simulink subsystem "sm_rc_initializer"  (R2023a)
settings: Solver=VariableStepAuto  StartTime=0.0  StopTime=10.0  RelTol=1e-3
settings Model: Creator=thesa  LastModifiedBy=thesa

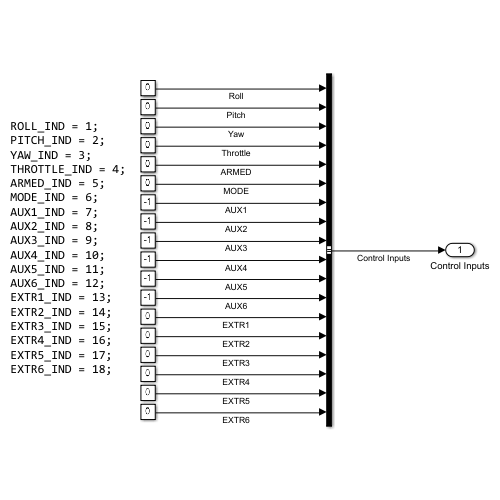
[thumbnail: Simulink's stored preview of the top-level diagram]
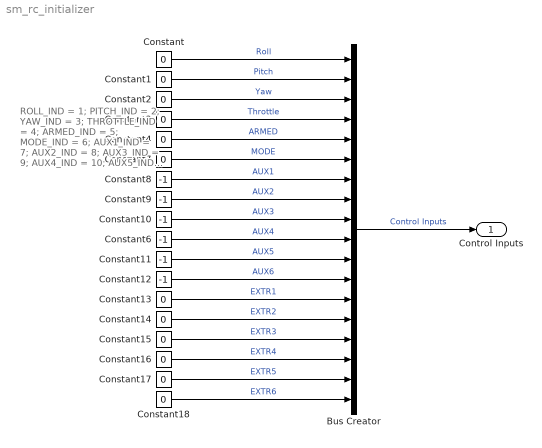
== system sm_rc_initializer ==
  note: ROLL_IND = 1;
      | PITCH_IND = 2;
      | YAW_IND = 3;
      | THROTTLE_IND = 4;
      | ARMED_IND = 5;
      | MODE_IND = 6;
      | AUX1_IND = 7;
      | AUX2_IND = 8;
      | AUX3_IND = 9;
      | AUX4_IND = 10;
      | AUX5_IND = 11;
      | AUX6_IND = 12;
      | EXTR1_IND = 13;
      | EXTR2_IND = 14;
      | EXTR3_IND = 15;
      | EXTR4_IND = 16;
      | EXTR5_IND = 17;
      | EXTR6_IND = 18;
  Bus Creator : BusCreator  Inputs=18
  Constant{,1..4,7,13..18} (12 alike) : Constant  Value=0
  Constant{6,8..12} (6 alike) : Constant  Value=-1
  Control Inputs : Outport
  wires:
  Constant12/1 -> Bus Creator/12  "AUX6"
  Constant8/1 -> Bus Creator/7  "AUX1"
  Constant16/1 -> Bus Creator/16  "EXTR4"
  Constant14/1 -> Bus Creator/14  "EXTR2"
  Constant13/1 -> Bus Creator/13  "EXTR1"
  Constant3/1 -> Bus Creator/4  "Throttle"
  Constant10/1 -> Bus Creator/9  "AUX3"
  Constant11/1 -> Bus Creator/11  "AUX5"
  Constant4/1 -> Bus Creator/5  "ARMED"
  Constant/1 -> Bus Creator/1  "Roll"
  Constant7/1 -> Bus Creator/6  "MODE"
  Constant2/1 -> Bus Creator/3  "Yaw"
  Constant18/1 -> Bus Creator/18  "EXTR6"
  Constant6/1 -> Bus Creator/10  "AUX4"
  Constant9/1 -> Bus Creator/8  "AUX2"
  Constant1/1 -> Bus Creator/2  "Pitch"
  Constant15/1 -> Bus Creator/15  "EXTR3"
  Constant17/1 -> Bus Creator/17  "EXTR5"
  Bus Creator/1 -> Control Inputs/1  "Control Inputs"
